simulink model "que6_2_sim"  (R2023a)
settings: Solver=VariableStepAuto  StartTime=0.0  StopTime=50  RelTol=1e-3
values from neighbouring files (symbols this model uses):
  A = [0 1 0 0 ... (first row only)    [que5_1.m]    (also in que5_1_1.m; que5_4.m; que6_1.m = [0 1 0; que6_2_sim_input.m = [0 1 0;0 0 1;0 0 -0.5])
  B = [0 ... (first row only)    [que5_1.m]    (also in que5_1_1.m; que5_4.m; que6_1.m = [0 0 0.5]'; que6_2_sim_input.m = [0;0;0.5])
  C = [1,0, 0, 0 ... (first row only)    [que5_1.m]    (also in que5_1_1.m; que5_4.m = [1, 0, 0, 0]; que6_1.m = [1 0 0; que6_2_sim_input.m = [1 0 0)
  D = [0]    [que5_4.m]    (also in que6_2_sim_input.m = [0; 0;0])
  K = place(A,B,P)    [que5_4.m]    (also in que6_2_sim_input.m = lqr(A,B,Q,R))
  K1 = lqr(A,B,Q,R2)    [que6_2_sim_input.m]
  K2 = lqr(A,B,Q2,R)    [que6_2_sim_input.m]
  K3 = lqr(A,B,Q3,R)    [que6_2_sim_input.m]
undefined symbols (not defined in the file or in its folder): Continuous, Time
libraries: ctrlSharedLib x4
settings Model: Creator=Hasee  LastModifiedBy=Administrator

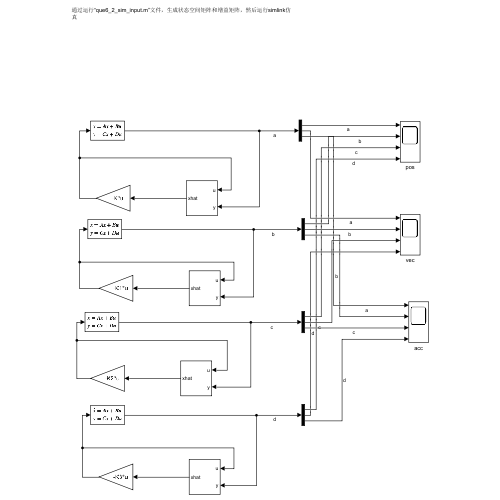
[thumbnail: Simulink's stored preview of the top-level diagram]
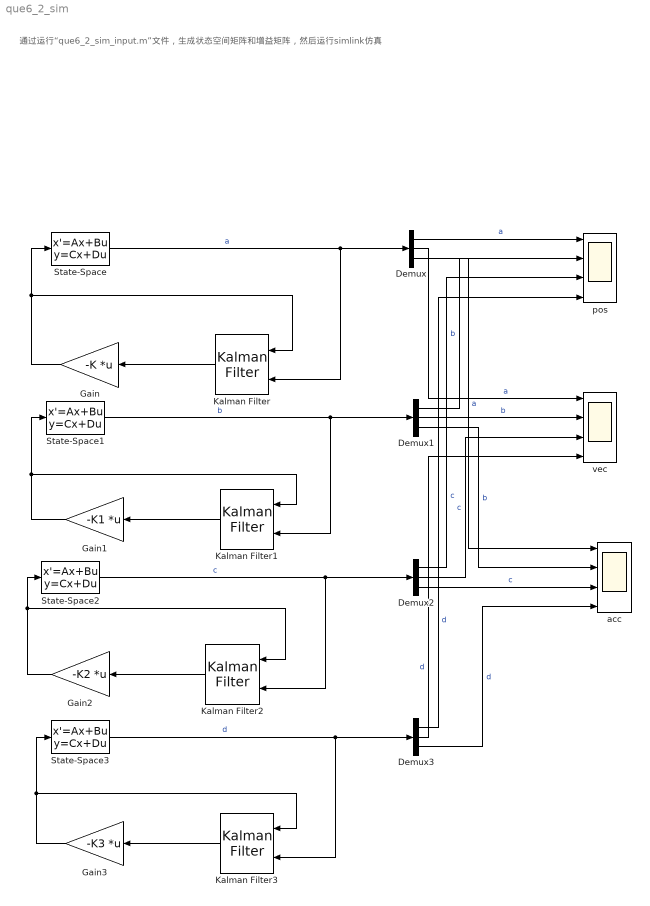
== system que6_2_sim ==
  note: 通过运行“que6_2_sim_input.m”文件，生成状态空间矩阵和增益矩阵，然后运行simlink仿真
  Demux{,1..3} (4 alike) : Demux  Outputs=3
  Gain : Gain  Gain=-K  Multiplication=Matrix(K*u)
  Gain1 : Gain  Gain=-K1  Multiplication=Matrix(K*u)
  Gain2 : Gain  Gain=-K2  Multiplication=Matrix(K*u)
  Gain3 : Gain  Gain=-K3  Multiplication=Matrix(K*u)
  Kalman Filter{,1..3} (4 alike) : ctrlSharedLib/Kalman Filter  TimeDomain=Continuous-Time  UseCurrentEstimator=on  ModelSource=Individual A, B, C, D matrices  ModelSourceVariable=ss(0.95,1,1,0,1)  A=A  B=B  C=C  D=D  NumberOfStates=1  NumberOfInputs=1  NumberOfOutputs=1  InitialEstimateSource=Dialog  X0=[10 0 0]  P0=10  UseK=off  UseGH=off  NumberOfProcessNoiseInputs=1  G=1  TimeInvariantG=on  H=0  TimeInvariantH=on  Q=0.05  TimeInvariantQ=on  R=1  TimeInvariantR=on  N=0  TimeInvariantN=on  AddInputPort=on  AddEnablePort=off  OutputEstimatedY=off  OutputP=off  Ts=-1
  State-Space{,1..3} (4 alike) : StateSpace  A=A  B=B  C=C  D=D  InitialCondition=[10 0 0]
  acc : Scope  NumInputPorts=4
  pos : Scope  NumInputPorts=4
  vec : Scope  NumInputPorts=4
  wires:
  Gain/1 -> State-Space/1, Kalman Filter/1
  Kalman Filter/1 -> Gain/1
  Gain1/1 -> State-Space1/1, Kalman Filter1/1
  Kalman Filter1/1 -> Gain1/1
  Gain2/1 -> State-Space2/1, Kalman Filter2/1
  Kalman Filter2/1 -> Gain2/1
  Gain3/1 -> State-Space3/1, Kalman Filter3/1
  Kalman Filter3/1 -> Gain3/1
  State-Space/1 -> Demux/1, Kalman Filter/2  "a"
  State-Space1/1 -> Demux1/1, Kalman Filter1/2  "b"
  State-Space2/1 -> Demux2/1, Kalman Filter2/2  "c"
  State-Space3/1 -> Demux3/1, Kalman Filter3/2  "d"
  Demux/1 -> pos/1  "a"
  Demux/2 -> vec/1  "a"
  Demux/3 -> acc/1  "a"
  Demux1/1 -> pos/2  "b"
  Demux1/2 -> vec/2  "b"
  Demux1/3 -> acc/2  "b"
  Demux2/1 -> pos/3  "c"
  Demux2/2 -> vec/3  "c"
  Demux2/3 -> acc/3  "c"
  Demux3/1 -> pos/4  "d"
  Demux3/2 -> vec/4  "d"
  Demux3/3 -> acc/4  "d"
